simulink model "abg_x_p"  (R2014b)
settings: Solver=ode3  StartTime=0.0  StopTime=simtime  FixedStep=0.001  RelTol=1e-3
values from neighbouring files (symbols this model uses):
  init_x_p = -9    [path_planning.m]    (also in path_planning_v0.m = -5; path_planning_v1.m = -9.9; path_planning_v2.m = 1; run.m = -5)
  init_x_p_dot = 0    [path_planning.m]    (also in path_planning_v0.m = 1; path_planning_v1.m = 1; path_planning_v2.m = 10; run.m)
  w = pi/10    (= 0.314159265359)    [path_config_cos.m]    (also in path_planning.m = 0.628318530718; path_planning_v0.m = 0.628318530718; path_planning_v1.m = 0.628318530718; path_planning_v2.m)
settings Model: Creator=Fredrik  LastModifiedBy=Fredrik

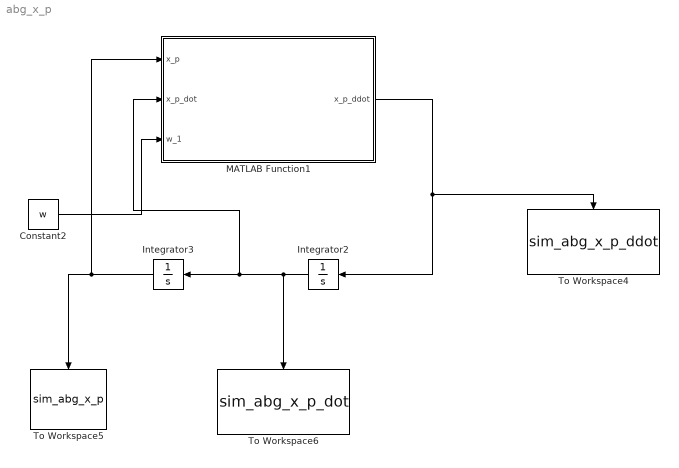
== system abg_x_p ==
  Constant2 : Constant  Value=w
  Integrator2 : Integrator  InitialCondition=init_x_p_dot
  Integrator3 : Integrator  InitialCondition=init_x_p
  MATLAB Function1 : MATLAB Function  TreatAsAtomicUnit=on
  To Workspace4 : ToWorkspace  VariableName=sim_abg_x_p_ddot  SaveFormat=Structure With Time  SampleTime=-1
  To Workspace5 : ToWorkspace  VariableName=sim_abg_x_p  SaveFormat=Structure With Time  SampleTime=-1
  To Workspace6 : ToWorkspace  VariableName=sim_abg_x_p_dot  SaveFormat=Structure With Time  SampleTime=-1
  wires:
  MATLAB Function1/1(x_p_ddot) -> To Workspace4/1, Integrator2/1
  Integrator3/1 -> MATLAB Function1/1(x_p), To Workspace5/1
  Integrator2/1 -> To Workspace6/1, MATLAB Function1/2(x_p_dot), Integrator3/1
  Constant2/1 -> MATLAB Function1/3(w_1)

== matlab function abg_x_p/MATLAB Function1 ==
  data: x_p input; x_p_ddot output; x_p_dot input; w_1 input
function x_p_ddot  = fcn(x_p, x_p_dot,w_1)
%#codegen

g=9.81;





%tanh
%alfa=a^3*tanh(w*x_p+b)^2*(1-tanh(w*x_p+b)^2)*w/sqrt(1-a^2*tanh(w*x_p+b)^2)-a^2*tanh(w*x_p+b)*(1-tanh(w*x_p+b)^2)*w/(sqrt(1-a^2*tanh(w*x_p+b)^2)*sqrt(a^2*tanh(w*x_p+b)^2));
%beta=a*tanh(w*x_p+b)*(a^4*tanh(w*x_p+b)^2*(1-tanh(w*x_p+b)^2)^2*w^2/(1-a^2*tanh(w*x_p+b)^2)^(3/2)+a^2*(1-tanh(w*x_p+b)^2)^2*w^2/sqrt(1-a^2*tanh(w*x_p+b)^2)-2*a^2*tanh(w*x_p+b)^2*(1-tanh(w*x_p+b)^2)*w^2/sqrt(1-a^2*tanh(w*x_p+b)^2))-a^4*tanh(w*x_p+b)^2*(1-tanh(w*x_p+b)^2)^2*w^2/((1-a^2*tanh(w*x_p+b)^2)^(3/2)*sqrt(a^2*tanh(w*x_p+b)^2))-a^2*(1-tanh(w*x_p+b)^2)^2*w^2/(sqrt(1-a^2*tanh(w*x_p+b)^2)*sqrt(a^2*tanh(w*x_p+b)^2))+2*a^2*tanh(w*x_p+b)^2*(1-tanh(w*x_p+b)^2)*w^2/(sqrt(1-a^2*tanh(w*x_p+b)^2)*sqrt(a^2*tanh(w*x_p+b)^2))+a^4*tanh(w*x_p+b)^2*(1-tanh(w*x_p+b)^2)^2*w^2/(sqrt(1-a^2*tanh(w*x_p+b)^2)*(a^2*tanh(w*x_p+b)^2)^(3/2));
%gamma=-g*sqrt(1-a^2*tanh(w*x_p+b)^2);



% cos switch

alfa=cos(w_1*x_p)*(1-cos(w_1*x_p)*w_1*sqrt(-cos(w_1*x_p)^2+1)/sqrt(sin(w_1*x_p)^2)+sin(w_1*x_p)^2*sqrt(-cos(w_1*x_p)^2+1)*cos(w_1*x_p)*w_1/(sin(w_1*x_p)^2)^(3/2)-sin(w_1*x_p)^2*cos(w_1*x_p)*w_1/(sqrt(sin(w_1*x_p)^2)*sqrt(-cos(w_1*x_p)^2+1)))+(-w_1*sqrt(-cos(w_1*x_p)^2+1)/sqrt(sin(w_1*x_p)^2)+sin(w_1*x_p)^2*sqrt(-cos(w_1*x_p)^2+1)*w_1/(sin(w_1*x_p)^2)^(3/2)-sin(w_1*x_p)^2*w_1/(sqrt(sin(w_1*x_p)^2)*sqrt(-cos(w_1*x_p)^2+1))-sin(w_1*x_p)^2*sqrt(-cos(w_1*x_p)^2+1)*w_1/(sqrt(sin(w_1*x_p)^2)*cos(w_1*x_p)^2))/(1+(-cos(w_1*x_p)^2+1)/cos(w_1*x_p)^2);
beta=cos(w_1*x_p)*(sin(w_1*x_p)*w_1^2*sqrt(-cos(w_1*x_p)^2+1)/sqrt(sin(w_1*x_p)^2)+3*cos(w_1*x_p)^2*w_1^2*sqrt(-cos(w_1*x_p)^2+1)*sin(w_1*x_p)/(sin(w_1*x_p)^2)^(3/2)-3*cos(w_1*x_p)^2*w_1^2*sin(w_1*x_p)/(sqrt(sin(w_1*x_p)^2)*sqrt(-cos(w_1*x_p)^2+1))-3*sin(w_1*x_p)^3*sqrt(-cos(w_1*x_p)^2+1)*cos(w_1*x_p)^2*w_1^2/(sin(w_1*x_p)^2)^(5/2)+2*sin(w_1*x_p)^3*cos(w_1*x_p)^2*w_1^2/((sin(w_1*x_p)^2)^(3/2)*sqrt(-cos(w_1*x_p)^2+1))-sin(w_1*x_p)^3*sqrt(-cos(w_1*x_p)^2+1)*w_1^2/(sin(w_1*x_p)^2)^(3/2)+sin(w_1*x_p)^3*cos(w_1*x_p)^2*w_1^2/(sqrt(sin(w_1*x_p)^2)*(-cos(w_1*x_p)^2+1)^(3/2))+sin(w_1*x_p)^3*w_1^2/(sqrt(sin(w_1*x_p)^2)*sqrt(-cos(w_1*x_p)^2+1)))+(3*w_1^2*sqrt(-cos(w_1*x_p)^2+1)*sin(w_1*x_p)*cos(w_1*x_p)/(sin(w_1*x_p)^2)^(3/2)-3*w_1^2*sin(w_1*x_p)*cos(w_1*x_p)/(sqrt(sin(w_1*x_p)^2)*sqrt(-cos(w_1*x_p)^2+1))-3*sin(w_1*x_p)^3*sqrt(-cos(w_1*x_p)^2+1)*w_1^2*cos(w_1*x_p)/(sin(w_1*x_p)^2)^(5/2)+2*sin(w_1*x_p)^3*w_1^2*cos(w_1*x_p)/((sin(w_1*x_p)^2)^(3/2)*sqrt(-cos(w_1*x_p)^2+1))+sin(w_1*x_p)^3*w_1^2*cos(w_1*x_p)/(sqrt(sin(w_1*x_p)^2)*(-cos(w_1*x_p)^2+1)^(3/2))-2*sin(w_1*x_p)*sqrt(-cos(w_1*x_p)^2+1)*w_1^2/(sqrt(sin(w_1*x_p)^2)*cos(w_1*x_p))+sin(w_1*x_p)^3*sqrt(-cos(w_1*x_p)^2+1)*w_1^2/((sin(w_1*x_p)^2)^(3/2)*cos(w_1*x_p))-sin(w_1*x_p)^3*w_1^2/(sqrt(sin(w_1*x_p)^2)*sqrt(-cos(w_1*x_p)^2+1)*cos(w_1*x_p))-2*sin(w_1*x_p)^3*sqrt(-cos(w_1*x_p)^2+1)*w_1^2/(sqrt(sin(w_1*x_p)^2)*cos(w_1*x_p)^3))/(1+(-cos(w_1*x_p)^2+1)/cos(w_1*x_p)^2)-(-w_1*sqrt(-cos(w_1*x_p)^2+1)/sqrt(sin(w_1*x_p)^2)+sin(w_1*x_p)^2*sqrt(-cos(w_1*x_p)^2+1)*w_1/(sin(w_1*x_p)^2)^(3/2)-sin(w_1*x_p)^2*w_1/(sqrt(sin(w_1*x_p)^2)*sqrt(-cos(w_1*x_p)^2+1))-sin(w_1*x_p)^2*sqrt(-cos(w_1*x_p)^2+1)*w_1/(sqrt(sin(w_1*x_p)^2)*cos(w_1*x_p)^2))*(2*sin(w_1*x_p)*w_1/cos(w_1*x_p)+(2*(-cos(w_1*x_p)^2+1))*sin(w_1*x_p)*w_1/cos(w_1*x_p)^3)/(1+(-cos(w_1*x_p)^2+1)/cos(w_1*x_p)^2)^2;
gamma=g*sin(w_1*x_p)*sqrt(-cos(w_1*x_p)^2+1)/sqrt(sin(w_1*x_p)^2);

x_p_ddot = (-beta*(x_p_dot^2) - gamma)/alfa;
